simulink model "IntegratedStarterGenerator_lithium_ion"  (R2024b)
settings: Solver=ode23tb  StartTime=0.0  StopTime=15  FixedStep=1e-6  RelTol=1e-4  EnableMultiTasking=on
PreLoadFcn:
  | BeltStarterGeneratorData;
model workspace (MAT data in the model file):
  Cdc = 0.001
  ID_MAP = [-155.095933536 -155.095933536 -155.095933536 -155.095933536 -155.095933536 -155.095933536 -155.095933536 -155.095933536 -200.847752045 -245.560073478 -288.511134519 -330.698372533 ... (48076 elements, 28x101x17)]
  IQ_MAP = [-234.678365656 -234.678365656 -234.678365656 -234.678365656 -234.678365656 -234.678365656 -234.678365656 -234.678365656 -207.892729616 -187.030522468 -170.586354015 -157.025794022 ... (48076 elements, 28x101x17)]
  Ki_dcdc = 10
  Ki_id = 170
  Ki_iq = 170
  Ki_vdc = 100
  Kp_dcdc = 0.5
  Kp_id = 0.24
  Kp_iq = 0.24
  Kp_vdc = 20
  L0 = 5e-05
  Ld = 0.00011
  Lq = 0.00011
  Pmax = 140
  RPM_VECT = [0 1000 2000 3000 4000 5000 6000 7000 8000 9000 10000]
  R_f : Simulink.Parameter (value not decoded)
  Rs = 0.085
  TQ_VECT = [-3.5 -3.43 -3.36 -3.29 -3.22 -3.15 -3.08 -3.01 -2.94 -2.87 -2.8 -2.73 ... (101 elements, 1x101)]
  Tmax = 3.5
  Ts = 5e-06
  Tsi = 0.0001
  VDC_VECT = [8 8.625 9.25 9.875 10.5 11.125 11.75 12.375 13 13.625 14.25 14.875 ... (17 elements, 1x17)]
  dend_id = [1 -0.966796355036]
  dend_iq = [1 -0.900395111642]
  fsw = 5000
  fswd = 5000
  numd_id = 0.0332036449638
  numd_iq = 0.099604888358
  p = 3
  psim = 0.0159
  r_tire : Simulink.Parameter (value not decoded)
  tout = [0 5e-06 1e-05 1.5e-05 2e-05 2.5e-05 3e-05 3.5e-05 4e-05 4.5e-05 5e-05 5.5e-05 ... (200005 elements, 200005x1)]
symbols that are objects in the model workspace (value not decoded): R_f, r_tire
undefined symbols (not defined in the file or in its folder): DiscIntNeverNeededParam
libraries: fl_lib x51, nesl_utility x26, simulink x12, ee_lib x6, eeDiscretePi x3, sdl_lib x2, eeTransforms x2, batteryecm_lib x1, eePmsmCurrentController x1, eePmsmCurrentReferenceGen x1, eePmsmTorqueEstimator x1, eePwmGeneratorTwoLevel x1
(part 3 of 3)

== system IntegratedStarterGenerator_lithium_ion/Thermal model/Sensing Temperature WiA ==
  PS-Simulink Converter : nesl_utility/PS-Simulink Converter  PhysicalDomain=network_engine_domain  SubClassName=ps_output  LeftPortType=input  RightPortType=output  PseudoPeriodic=off  Frequencies=[]  VectorFormat=1-D array  Unit=degC  AffineConversion=on
  Temperature Sensor : fl_lib/Thermal/Thermal Sensors/Temperature Sensor  temperature_measure=foundation.enum.MeasurementReference.difference
  ThRef : fl_lib/Thermal/Thermal Elements/Thermal Reference
  H : PMIOPort  Side=Left
  tag scope: TA=global
  wires:
  PS-Simulink Converter/1 -> [TA]
  connections:
  H/RConn1 -- Temperature Sensor/LConn1
  ThRef/LConn1 -- Temperature Sensor/RConn1
  Temperature Sensor/RConn2 -- PS-Simulink Converter/LConn1

== system IntegratedStarterGenerator_lithium_ion/Thermal model/Sensing Temperature WiB ==
  PS-Simulink Converter : nesl_utility/PS-Simulink Converter  PhysicalDomain=network_engine_domain  SubClassName=ps_output  LeftPortType=input  RightPortType=output  PseudoPeriodic=off  Frequencies=[]  VectorFormat=1-D array  Unit=degC  AffineConversion=on
  Temperature Sensor : fl_lib/Thermal/Thermal Sensors/Temperature Sensor  temperature_measure=foundation.enum.MeasurementReference.difference
  ThRef : fl_lib/Thermal/Thermal Elements/Thermal Reference
  H : PMIOPort  Side=Left
  tag scope: TB=global
  wires:
  PS-Simulink Converter/1 -> [TB]
  connections:
  Temperature Sensor/RConn2 -- PS-Simulink Converter/LConn1
  ThRef/LConn1 -- Temperature Sensor/RConn1
  H/RConn1 -- Temperature Sensor/LConn1

== system IntegratedStarterGenerator_lithium_ion/Thermal model/Sensing Temperature WiC ==
  PS-Simulink Converter : nesl_utility/PS-Simulink Converter  PhysicalDomain=network_engine_domain  SubClassName=ps_output  LeftPortType=input  RightPortType=output  PseudoPeriodic=off  Frequencies=[]  VectorFormat=1-D array  Unit=degC  AffineConversion=on
  Temperature Sensor : fl_lib/Thermal/Thermal Sensors/Temperature Sensor  temperature_measure=foundation.enum.MeasurementReference.difference
  ThRef : fl_lib/Thermal/Thermal Elements/Thermal Reference
  H : PMIOPort  Side=Left
  tag scope: TC=global
  wires:
  PS-Simulink Converter/1 -> [TC]
  connections:
  H/RConn1 -- Temperature Sensor/LConn1
  ThRef/LConn1 -- Temperature Sensor/RConn1
  Temperature Sensor/RConn2 -- PS-Simulink Converter/LConn1

== system IntegratedStarterGenerator_lithium_ion/EM Controller/Measurements/Vdc Filter ==
  In : Inport
  Discrete Transfer Fcn : DiscreteTransferFcn  Numerator=num  Denominator=den
  Out : Outport  VectorParamsAs1DForOutWhenUnconnected=off
  wires:
  In/1 -> Discrete Transfer Fcn/1
  Discrete Transfer Fcn/1 -> Out/1

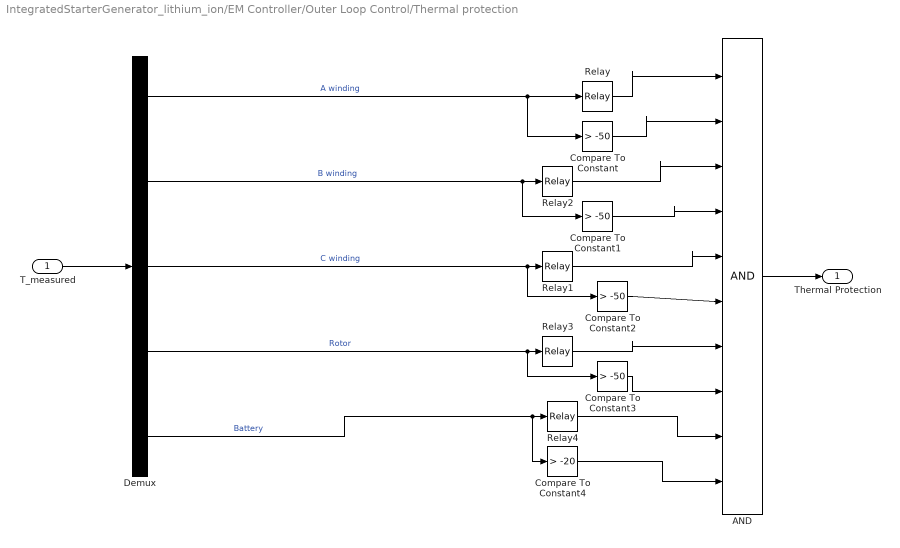
== system IntegratedStarterGenerator_lithium_ion/EM Controller/Outer Loop Control/Thermal protection ==
  T_measured : Inport
  AND : Logic  Inputs=10  IconShape=distinctive  AllPortsSameDT=off  OutDataTypeStr=boolean
  Compare To Constant{,1..3} (4 alike) : simulink/Logic and Bit Operations/Compare To Constant  relop=>  const=-50  OutDataTypeStr=boolean  ZeroCross=off
  Compare To Constant4 : simulink/Logic and Bit Operations/Compare To Constant  relop=>  const=-20  OutDataTypeStr=boolean  ZeroCross=off
  Demux : Demux  Outputs=5
  Relay{,1..3} (4 alike) : Relay  OnSwitchValue=120  OffSwitchValue=80  OnOutputValue=0  OffOutputValue=1  ZeroCross=off
  Relay4 : Relay  OnSwitchValue=50  OffSwitchValue=36  OnOutputValue=0  OffOutputValue=1  ZeroCross=off
  Thermal Protection : Outport
  wires:
  Demux/5 -> Compare To Constant4/1, Relay4/1  "Battery"
  Demux/4 -> Compare To Constant3/1, Relay3/1  "Rotor"
  Demux/3 -> Compare To Constant2/1, Relay1/1  "C winding"
  Demux/2 -> Compare To Constant1/1, Relay2/1  "B winding"
  Demux/1 -> Compare To Constant/1, Relay/1  "A winding"
  Relay/1 -> AND/1
  AND/1 -> Thermal Protection/1
  T_measured/1 -> Demux/1
  Relay2/1 -> AND/3
  Relay1/1 -> AND/5
  Relay3/1 -> AND/7
  Relay4/1 -> AND/9
  Compare To Constant/1 -> AND/2
  Compare To Constant1/1 -> AND/4
  Compare To Constant2/1 -> AND/6
  Compare To Constant3/1 -> AND/8
  Compare To Constant4/1 -> AND/10

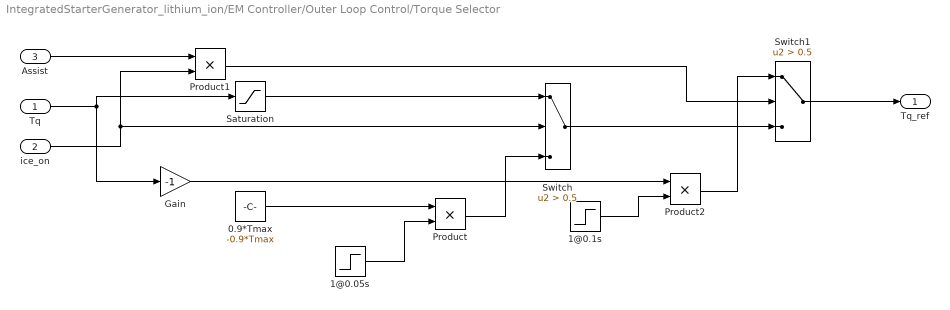
== system IntegratedStarterGenerator_lithium_ion/EM Controller/Outer Loop Control/Torque Selector ==
  Tq : Inport
  ice_on : Inport  Port=2
  Assist : Inport  Port=3
  0.9*Tmax : Constant  Value=-0.9*Tmax  SampleTime=-1
  1@0.05s : Step  Time=0.05  ZeroCross=off
  1@0.1s : Step  Time=0.1  ZeroCross=off
  Gain : Gain  Gain=-1
  Product : Product
  Product1 : Product
  Product2 : Product
  Saturation : Saturate  UpperLimit=Tmax  LowerLimit=-Tmax
  Switch : Switch  Criteria=u2 > Threshold  Threshold=0.5  ZeroCross=off  SaturateOnIntegerOverflow=off  InputSameDT=off
  Switch1 : Switch  Criteria=u2 > Threshold  Threshold=0.5  ZeroCross=off  SaturateOnIntegerOverflow=off  InputSameDT=off
  Tq_ref : Outport  VectorParamsAs1DForOutWhenUnconnected=off
  wires:
  Tq/1 -> Gain/1, Saturation/1
  ice_on/1 -> Product1/2, Switch/2
  1@0.05s/1 -> Product/2
  0.9*Tmax/1 -> Product/1
  Product/1 -> Switch/3
  Assist/1 -> Product1/1
  Product1/1 -> Switch1/2
  1@0.1s/1 -> Product2/2
  Switch/1 -> Switch1/3
  Product2/1 -> Switch1/1
  Gain/1 -> Product2/1
  Saturation/1 -> Switch/1
  Switch1/1 -> Tq_ref/1

== stateflow chart IntegratedStarterGenerator_lithium_ion/EM Controller/Task Scheduler ==
  (default) -> (junction 105) : CLK_50us
  (junction 105) -> (junction 106)
  (junction 106) -> (junction 112) [order 2]
  (junction 106) -> (junction 112) [order 1] : [cnt%%2==0]{Task_100us_1;}
  (junction 112) -> (junction 110) [order 2]
  (junction 112) -> (junction 110) [order 1] : [cnt%%2==0]{Task_100us_2;}
  (junction 110) -> (junction 111) [order 2]
  (junction 110) -> (junction 111) [order 1] : [cnt%%20==0]{Task_1ms_1;}
  (junction 111) -> (junction 107) [order 2]
  (junction 111) -> (junction 108) [order 1] : [1]{cnt++;}
  data: cnt local int32
  events: Task_100us_1 output FUNCTION_CALL_EVENT; Task_100us_2 output FUNCTION_CALL_EVENT; Task_1ms_1 output FUNCTION_CALL_EVENT; CLK_50us input FUNCTION_CALL_EVENT

== matlab function IntegratedStarterGenerator_lithium_ion/MATLAB Function ==
  data: V_kmph input; gear_ratio output
% MATLAB Function block: CVT_Gear_Calculation
% Inputs: V_kmph (vehicle speed in km/h)
% Output: gear_ratio
function gear_ratio = fcn(V_kmph)
    % Define piecewise gear ratio logic based on vehicle speed
    if V_kmph <= 10
        gear_ratio = 4.0;
    elseif V_kmph <= 20
        gear_ratio = 3.5;
    elseif V_kmph <= 30
        gear_ratio = 2.5;
    elseif V_kmph <= 40
        gear_ratio = 1.8;
    else
        gear_ratio = 1.5; % top gear
    end
end
